simulink model "DconstI_snt"  (R2025b)
settings: Solver=ode45  StartTime=0.0  StopTime=10.0  RelTol=1e-3  EnableMultiTasking=on
undefined symbols (not defined in the file or in its folder): DiscIntNeverNeededParam, Ts
libraries: fl_lib x12, nesl_utility x12, mcbeeMathTransformLib x12, eeTransforms x12
settings Model: Creator=gdudgeon  LastModifiedBy=gdudgeon
settings SolverCC: AlgebraicLoopSolver=TrustRegion
settings DataIOCC: LimitDataPoints=on  SaveFormat=Array  ReturnWorkspaceOutputs=off
settings OptimizationCC: ExpressionDepthLimit=2147483647.0  LifeSpan=inf
settings DebuggingCC: UnderspecifiedInitializationDetection=Classic  MergeDetectMultiDrivingBlocksExec=none  SolverPrmCheckMsg=warning  UnconnectedInputMsg=warning  UnconnectedOutputMsg=warning  UnconnectedLineMsg=warning  StateNameClashWarn=warning  SFUnexpectedBacktrackingDiag=warning  SFNoUnconditionalDefaultTransitionDiag=warning  SFExecutionAtInitializationDiag=none  ArithmeticOperatorsInVariantConditions=warning
settings HardwareCC: ProdBitPerPointer=32.0  ProdBitPerSizeT=32.0  ProdBitPerPtrDiffT=32.0  ProdLargestAtomicFloat=None  ProdIntDivRoundTo=Undefined  ProdEndianess=Unspecified  ProdWordSize=32.0  ProdHWDeviceType=32-bit Generic
settings ModelReferenceCC: EnableRefExpFcnMdlSchedulingChecks=on  PropagateSignalLabelsOutOfModel=off
settings SFSimCC: SimUseLocalCustomCode=off  CustomCodeUndefinedFunction=UseInterfaceOnly
settings RTWCC: RTWUseLocalCustomCode=off  GPUComputeCapability=3.5
settings CodeAppCC: StateflowObjectComments=on
settings GRTTargetCC: TargetLangStandard=C89/C90 (ANSI)
settings ConfigComp: CovMetricSettings=dw  CovSaveCumulativeToWorkspaceVar=on  CovSaveSingleToWorkspaceVar=on  CovExternalEMLEnable=off  CovSFcnEnable=off
settings SimscapeCC: SimscapeNormalizeSystem=off

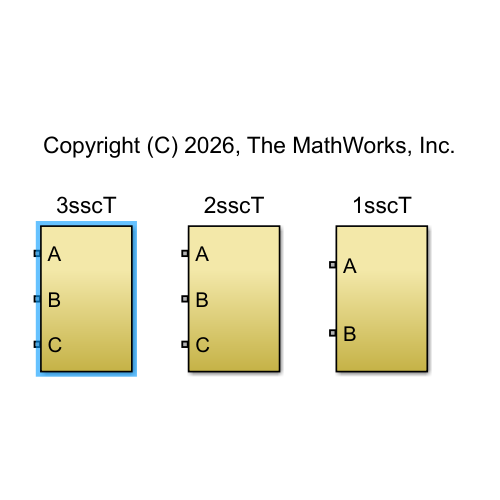
[thumbnail: Simulink's stored preview of the top-level diagram]
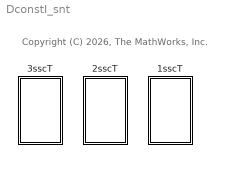
== system DconstI_snt ==
  note: Copyright (C) 2026, The MathWorks, Inc.
  1sscT : Subsystem
  2sscT : Subsystem
  3sscT : Subsystem

== system DconstI_snt/1sscT ==
  PQ1 : From
  constI1 : Subsystem  mask{V=4160*sqrt(2)}
      mask prompts: V "Vpk (V)"
  A : PMIOPort  Side=Left
  B : PMIOPort  Port=2  Side=Left
  wires:
  PQ1/1 -> constI1/1(PQ)
  connections:
  constI1/RConn1 -- A/RConn1
  constI1/LConn1 -- B/RConn1

== system DconstI_snt/2sscT ==
  PQ1 : From
  PQ2 : From
  constI1 : Subsystem  mask{V=4160*sqrt(2)}
      mask prompts: V "Vpk (V)"
  constI2 : Subsystem  mask{V=4160*sqrt(2)}
      mask prompts: V "Vpk (V)"
  A : PMIOPort  Side=Left
  B : PMIOPort  Port=2  Side=Left
  C : PMIOPort  Port=3  Side=Left
  wires:
  PQ2/1 -> constI2/1(PQ)
  PQ1/1 -> constI1/1(PQ)
  connections:
  constI2/LConn1 -- C/RConn1
  B/RConn1 -- constI2/RConn1 -- constI1/LConn1
  constI1/RConn1 -- A/RConn1

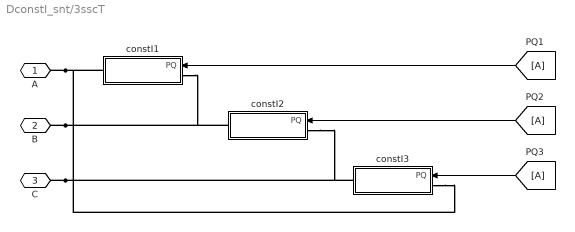
== system DconstI_snt/3sscT ==
  PQ1 : From
  PQ2 : From
  PQ3 : From
  constI1 : Subsystem  mask{V=4160*sqrt(2)}
      mask prompts: V "Vpk (V)"
  constI2 : Subsystem  mask{V=4160*sqrt(2)}
      mask prompts: V "Vpk (V)"
  constI3 : Subsystem  mask{V=4160*sqrt(2)}
      mask prompts: V "Vpk (V)"
  A : PMIOPort  Side=Left
  B : PMIOPort  Port=2  Side=Left
  C : PMIOPort  Port=3  Side=Left
  wires:
  PQ3/1 -> constI3/1(PQ)
  PQ1/1 -> constI1/1(PQ)
  PQ2/1 -> constI2/1(PQ)
  connections:
  A/RConn1 -- constI3/LConn1 -- constI1/RConn1
  B/RConn1 -- constI2/RConn1 -- constI1/LConn1
  C/RConn1 -- constI3/RConn1 -- constI2/LConn1

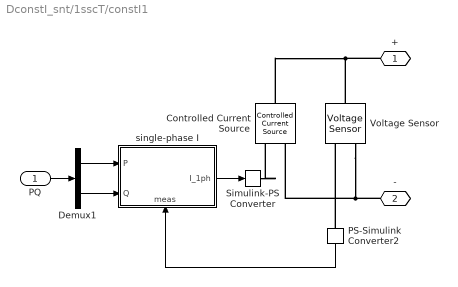
== system DconstI_snt/1sscT/constI1 ==
  PQ : Inport
  Controlled Current Source : fl_lib/Electrical/Electrical Sources/Controlled Current Source
  Demux1 : Demux  Outputs=2
  PS-Simulink Converter2 : nesl_utility/PS-Simulink Converter  PhysicalDomain=network_engine_domain  SubClassName=ps_output  LeftPortType=input  RightPortType=output  PseudoPeriodic=off  Frequencies=[]  VectorFormat=inherit  Unit=inherit  AffineConversion=off
  Simulink-PS Converter : nesl_utility/Simulink-PS Converter  PhysicalDomain=network_engine_domain  SubClassName=ps_input  LeftPortType=input  RightPortType=output  PseudoPeriodic=off  Frequencies=[]  NoiseDistribution=none  NoiseParameters=[]  Unit=1  AffineConversion=off  FilteringAndDerivatives=zero  SimscapeFilterOrder=1  InputFilterTimeConstant=0.001  UdotUserProvided=0
  Voltage Sensor : fl_lib/Electrical/Electrical Sensors/Voltage Sensor
  single-phase I : Subsystem
      settings: PortSchema="{\"entries\":[{\"content\":{\"sides\":[{\"content\":{\"connectorIds\":[\"In1\",\"In2\"]},\"type\":\"ConnectorPlacement.EquallySpacedRectSide\",\"uuid\":\"dcb77ad6-d65a-4afe-9b75-44cea2e03bc8\"},{\"content\":{\"connectorIds\":[\"Out1\"],\"side\":\"RIGHT\"},\"type\":\"ConnectorPlacement.EquallySpacedRectSide\",\"uuid\":\"20550ec8-912f-4e6b-8efc-55d7f6680ac4\"},{\"content\":{\"side\":\"TOP\"},\"type\":\"ConnectorPlacement.EquallySpacedRectSide\",\"uuid\":\"6ad8cbf4-1495-4620-97d9-4b8af34d00d1\"},{\"content\":{\"connectorIds\":[\"In3\"],\"side\":\"BOTTOM\"},\"type\":\"ConnectorPlacement.EquallySpacedRectSide\",\"uuid\":\"0b9a8788-8400-4a69-9d07-dd0028530e33\"}]},\"type\":\"ConnectorPlacement.EquallySpacedConnector\",\"uuid\":\"b57ec49b-aa32-43b3-a026-14ed90072d63\"}],\"packageUris\":[\"http://schema.mathworks.com/mf0/Connector/R2020b\"],\"version\":\"1.0\"}"
  + : PMIOPort  Side=Right
  - : PMIOPort  Port=2  Side=Left
  wires:
  single-phase I/1(I_1ph) -> Simulink-PS Converter/1
  Demux1/1 -> single-phase I/1(P)
  PQ/1 -> Demux1/1
  PS-Simulink Converter2/1 -> single-phase I/3(meas)
  Demux1/2 -> single-phase I/2(Q)
  connections:
  PS-Simulink Converter2/LConn1 -- Voltage Sensor/RConn1
  Simulink-PS Converter/RConn1 -- Controlled Current Source/RConn1
  -/RConn1 -- Controlled Current Source/RConn2 -- Voltage Sensor/RConn2
  +/RConn1 -- Controlled Current Source/LConn1 -- Voltage Sensor/LConn1

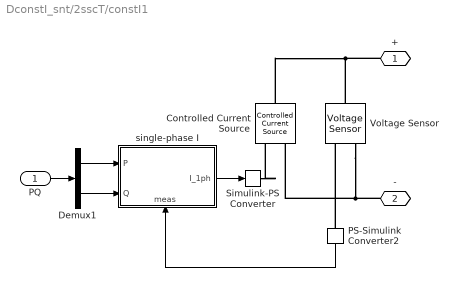
== system DconstI_snt/2sscT/constI1 ==
  PQ : Inport
  Controlled Current Source : fl_lib/Electrical/Electrical Sources/Controlled Current Source
  Demux1 : Demux  Outputs=2
  PS-Simulink Converter2 : nesl_utility/PS-Simulink Converter  PhysicalDomain=network_engine_domain  SubClassName=ps_output  LeftPortType=input  RightPortType=output  PseudoPeriodic=off  Frequencies=[]  VectorFormat=inherit  Unit=inherit  AffineConversion=off
  Simulink-PS Converter : nesl_utility/Simulink-PS Converter  PhysicalDomain=network_engine_domain  SubClassName=ps_input  LeftPortType=input  RightPortType=output  PseudoPeriodic=off  Frequencies=[]  NoiseDistribution=none  NoiseParameters=[]  Unit=1  AffineConversion=off  FilteringAndDerivatives=zero  SimscapeFilterOrder=1  InputFilterTimeConstant=0.001  UdotUserProvided=0
  Voltage Sensor : fl_lib/Electrical/Electrical Sensors/Voltage Sensor
  single-phase I : Subsystem
      settings: PortSchema="{\"entries\":[{\"content\":{\"sides\":[{\"content\":{\"connectorIds\":[\"In1\",\"In2\"]},\"type\":\"ConnectorPlacement.EquallySpacedRectSide\",\"uuid\":\"dcb77ad6-d65a-4afe-9b75-44cea2e03bc8\"},{\"content\":{\"connectorIds\":[\"Out1\"],\"side\":\"RIGHT\"},\"type\":\"ConnectorPlacement.EquallySpacedRectSide\",\"uuid\":\"20550ec8-912f-4e6b-8efc-55d7f6680ac4\"},{\"content\":{\"side\":\"TOP\"},\"type\":\"ConnectorPlacement.EquallySpacedRectSide\",\"uuid\":\"6ad8cbf4-1495-4620-97d9-4b8af34d00d1\"},{\"content\":{\"connectorIds\":[\"In3\"],\"side\":\"BOTTOM\"},\"type\":\"ConnectorPlacement.EquallySpacedRectSide\",\"uuid\":\"0b9a8788-8400-4a69-9d07-dd0028530e33\"}]},\"type\":\"ConnectorPlacement.EquallySpacedConnector\",\"uuid\":\"b57ec49b-aa32-43b3-a026-14ed90072d63\"}],\"packageUris\":[\"http://schema.mathworks.com/mf0/Connector/R2020b\"],\"version\":\"1.0\"}"
  + : PMIOPort  Side=Right
  - : PMIOPort  Port=2  Side=Left
  wires:
  single-phase I/1(I_1ph) -> Simulink-PS Converter/1
  Demux1/1 -> single-phase I/1(P)
  PQ/1 -> Demux1/1
  PS-Simulink Converter2/1 -> single-phase I/3(meas)
  Demux1/2 -> single-phase I/2(Q)
  connections:
  PS-Simulink Converter2/LConn1 -- Voltage Sensor/RConn1
  Simulink-PS Converter/RConn1 -- Controlled Current Source/RConn1
  -/RConn1 -- Controlled Current Source/RConn2 -- Voltage Sensor/RConn2
  +/RConn1 -- Controlled Current Source/LConn1 -- Voltage Sensor/LConn1

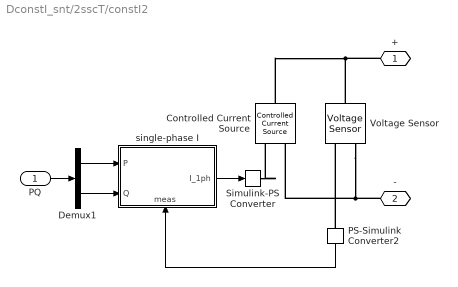
== system DconstI_snt/2sscT/constI2 ==
  PQ : Inport
  Controlled Current Source : fl_lib/Electrical/Electrical Sources/Controlled Current Source
  Demux1 : Demux  Outputs=2
  PS-Simulink Converter2 : nesl_utility/PS-Simulink Converter  PhysicalDomain=network_engine_domain  SubClassName=ps_output  LeftPortType=input  RightPortType=output  PseudoPeriodic=off  Frequencies=[]  VectorFormat=inherit  Unit=inherit  AffineConversion=off
  Simulink-PS Converter : nesl_utility/Simulink-PS Converter  PhysicalDomain=network_engine_domain  SubClassName=ps_input  LeftPortType=input  RightPortType=output  PseudoPeriodic=off  Frequencies=[]  NoiseDistribution=none  NoiseParameters=[]  Unit=1  AffineConversion=off  FilteringAndDerivatives=zero  SimscapeFilterOrder=1  InputFilterTimeConstant=0.001  UdotUserProvided=0
  Voltage Sensor : fl_lib/Electrical/Electrical Sensors/Voltage Sensor
  single-phase I : Subsystem
      settings: PortSchema="{\"entries\":[{\"content\":{\"sides\":[{\"content\":{\"connectorIds\":[\"In1\",\"In2\"]},\"type\":\"ConnectorPlacement.EquallySpacedRectSide\",\"uuid\":\"dcb77ad6-d65a-4afe-9b75-44cea2e03bc8\"},{\"content\":{\"connectorIds\":[\"Out1\"],\"side\":\"RIGHT\"},\"type\":\"ConnectorPlacement.EquallySpacedRectSide\",\"uuid\":\"20550ec8-912f-4e6b-8efc-55d7f6680ac4\"},{\"content\":{\"side\":\"TOP\"},\"type\":\"ConnectorPlacement.EquallySpacedRectSide\",\"uuid\":\"6ad8cbf4-1495-4620-97d9-4b8af34d00d1\"},{\"content\":{\"connectorIds\":[\"In3\"],\"side\":\"BOTTOM\"},\"type\":\"ConnectorPlacement.EquallySpacedRectSide\",\"uuid\":\"0b9a8788-8400-4a69-9d07-dd0028530e33\"}]},\"type\":\"ConnectorPlacement.EquallySpacedConnector\",\"uuid\":\"b57ec49b-aa32-43b3-a026-14ed90072d63\"}],\"packageUris\":[\"http://schema.mathworks.com/mf0/Connector/R2020b\"],\"version\":\"1.0\"}"
  + : PMIOPort  Side=Right
  - : PMIOPort  Port=2  Side=Left
  wires:
  Demux1/2 -> single-phase I/2(Q)
  PS-Simulink Converter2/1 -> single-phase I/3(meas)
  PQ/1 -> Demux1/1
  Demux1/1 -> single-phase I/1(P)
  single-phase I/1(I_1ph) -> Simulink-PS Converter/1
  connections:
  Voltage Sensor/LConn1 -- Controlled Current Source/LConn1 -- +/RConn1
  Voltage Sensor/RConn2 -- Controlled Current Source/RConn2 -- -/RConn1
  Simulink-PS Converter/RConn1 -- Controlled Current Source/RConn1
  PS-Simulink Converter2/LConn1 -- Voltage Sensor/RConn1

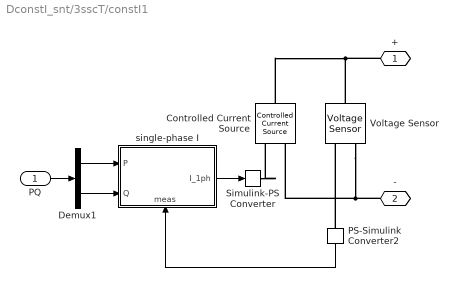
== system DconstI_snt/3sscT/constI1 ==
  PQ : Inport
  Controlled Current Source : fl_lib/Electrical/Electrical Sources/Controlled Current Source
  Demux1 : Demux  Outputs=2
  PS-Simulink Converter2 : nesl_utility/PS-Simulink Converter  PhysicalDomain=network_engine_domain  SubClassName=ps_output  LeftPortType=input  RightPortType=output  PseudoPeriodic=off  Frequencies=[]  VectorFormat=inherit  Unit=inherit  AffineConversion=off
  Simulink-PS Converter : nesl_utility/Simulink-PS Converter  PhysicalDomain=network_engine_domain  SubClassName=ps_input  LeftPortType=input  RightPortType=output  PseudoPeriodic=off  Frequencies=[]  NoiseDistribution=none  NoiseParameters=[]  Unit=1  AffineConversion=off  FilteringAndDerivatives=zero  SimscapeFilterOrder=1  InputFilterTimeConstant=0.001  UdotUserProvided=0
  Voltage Sensor : fl_lib/Electrical/Electrical Sensors/Voltage Sensor
  single-phase I : Subsystem
      settings: PortSchema="{\"entries\":[{\"content\":{\"sides\":[{\"content\":{\"connectorIds\":[\"In1\",\"In2\"]},\"type\":\"ConnectorPlacement.EquallySpacedRectSide\",\"uuid\":\"dcb77ad6-d65a-4afe-9b75-44cea2e03bc8\"},{\"content\":{\"connectorIds\":[\"Out1\"],\"side\":\"RIGHT\"},\"type\":\"ConnectorPlacement.EquallySpacedRectSide\",\"uuid\":\"20550ec8-912f-4e6b-8efc-55d7f6680ac4\"},{\"content\":{\"side\":\"TOP\"},\"type\":\"ConnectorPlacement.EquallySpacedRectSide\",\"uuid\":\"6ad8cbf4-1495-4620-97d9-4b8af34d00d1\"},{\"content\":{\"connectorIds\":[\"In3\"],\"side\":\"BOTTOM\"},\"type\":\"ConnectorPlacement.EquallySpacedRectSide\",\"uuid\":\"0b9a8788-8400-4a69-9d07-dd0028530e33\"}]},\"type\":\"ConnectorPlacement.EquallySpacedConnector\",\"uuid\":\"b57ec49b-aa32-43b3-a026-14ed90072d63\"}],\"packageUris\":[\"http://schema.mathworks.com/mf0/Connector/R2020b\"],\"version\":\"1.0\"}"
  + : PMIOPort  Side=Right
  - : PMIOPort  Port=2  Side=Left
  wires:
  single-phase I/1(I_1ph) -> Simulink-PS Converter/1
  Demux1/1 -> single-phase I/1(P)
  PQ/1 -> Demux1/1
  PS-Simulink Converter2/1 -> single-phase I/3(meas)
  Demux1/2 -> single-phase I/2(Q)
  connections:
  PS-Simulink Converter2/LConn1 -- Voltage Sensor/RConn1
  Simulink-PS Converter/RConn1 -- Controlled Current Source/RConn1
  -/RConn1 -- Controlled Current Source/RConn2 -- Voltage Sensor/RConn2
  +/RConn1 -- Controlled Current Source/LConn1 -- Voltage Sensor/LConn1

== system DconstI_snt/3sscT/constI2 ==
  PQ : Inport
  Controlled Current Source : fl_lib/Electrical/Electrical Sources/Controlled Current Source
  Demux1 : Demux  Outputs=2
  PS-Simulink Converter2 : nesl_utility/PS-Simulink Converter  PhysicalDomain=network_engine_domain  SubClassName=ps_output  LeftPortType=input  RightPortType=output  PseudoPeriodic=off  Frequencies=[]  VectorFormat=inherit  Unit=inherit  AffineConversion=off
  Simulink-PS Converter : nesl_utility/Simulink-PS Converter  PhysicalDomain=network_engine_domain  SubClassName=ps_input  LeftPortType=input  RightPortType=output  PseudoPeriodic=off  Frequencies=[]  NoiseDistribution=none  NoiseParameters=[]  Unit=1  AffineConversion=off  FilteringAndDerivatives=zero  SimscapeFilterOrder=1  InputFilterTimeConstant=0.001  UdotUserProvided=0
  Voltage Sensor : fl_lib/Electrical/Electrical Sensors/Voltage Sensor
  single-phase I : Subsystem
      settings: PortSchema="{\"entries\":[{\"content\":{\"sides\":[{\"content\":{\"connectorIds\":[\"In1\",\"In2\"]},\"type\":\"ConnectorPlacement.EquallySpacedRectSide\",\"uuid\":\"dcb77ad6-d65a-4afe-9b75-44cea2e03bc8\"},{\"content\":{\"connectorIds\":[\"Out1\"],\"side\":\"RIGHT\"},\"type\":\"ConnectorPlacement.EquallySpacedRectSide\",\"uuid\":\"20550ec8-912f-4e6b-8efc-55d7f6680ac4\"},{\"content\":{\"side\":\"TOP\"},\"type\":\"ConnectorPlacement.EquallySpacedRectSide\",\"uuid\":\"6ad8cbf4-1495-4620-97d9-4b8af34d00d1\"},{\"content\":{\"connectorIds\":[\"In3\"],\"side\":\"BOTTOM\"},\"type\":\"ConnectorPlacement.EquallySpacedRectSide\",\"uuid\":\"0b9a8788-8400-4a69-9d07-dd0028530e33\"}]},\"type\":\"ConnectorPlacement.EquallySpacedConnector\",\"uuid\":\"b57ec49b-aa32-43b3-a026-14ed90072d63\"}],\"packageUris\":[\"http://schema.mathworks.com/mf0/Connector/R2020b\"],\"version\":\"1.0\"}"
  + : PMIOPort  Side=Right
  - : PMIOPort  Port=2  Side=Left
  wires:
  Demux1/2 -> single-phase I/2(Q)
  PS-Simulink Converter2/1 -> single-phase I/3(meas)
  PQ/1 -> Demux1/1
  Demux1/1 -> single-phase I/1(P)
  single-phase I/1(I_1ph) -> Simulink-PS Converter/1
  connections:
  Voltage Sensor/LConn1 -- Controlled Current Source/LConn1 -- +/RConn1
  Voltage Sensor/RConn2 -- Controlled Current Source/RConn2 -- -/RConn1
  Simulink-PS Converter/RConn1 -- Controlled Current Source/RConn1
  PS-Simulink Converter2/LConn1 -- Voltage Sensor/RConn1

== system DconstI_snt/3sscT/constI3 ==
  PQ : Inport
  Controlled Current Source : fl_lib/Electrical/Electrical Sources/Controlled Current Source
  Demux1 : Demux  Outputs=2
  PS-Simulink Converter2 : nesl_utility/PS-Simulink Converter  PhysicalDomain=network_engine_domain  SubClassName=ps_output  LeftPortType=input  RightPortType=output  PseudoPeriodic=off  Frequencies=[]  VectorFormat=inherit  Unit=inherit  AffineConversion=off
  Simulink-PS Converter : nesl_utility/Simulink-PS Converter  PhysicalDomain=network_engine_domain  SubClassName=ps_input  LeftPortType=input  RightPortType=output  PseudoPeriodic=off  Frequencies=[]  NoiseDistribution=none  NoiseParameters=[]  Unit=1  AffineConversion=off  FilteringAndDerivatives=zero  SimscapeFilterOrder=1  InputFilterTimeConstant=0.001  UdotUserProvided=0
  Voltage Sensor : fl_lib/Electrical/Electrical Sensors/Voltage Sensor
  single-phase I : Subsystem
      settings: PortSchema="{\"entries\":[{\"content\":{\"sides\":[{\"content\":{\"connectorIds\":[\"In1\",\"In2\"]},\"type\":\"ConnectorPlacement.EquallySpacedRectSide\",\"uuid\":\"dcb77ad6-d65a-4afe-9b75-44cea2e03bc8\"},{\"content\":{\"connectorIds\":[\"Out1\"],\"side\":\"RIGHT\"},\"type\":\"ConnectorPlacement.EquallySpacedRectSide\",\"uuid\":\"20550ec8-912f-4e6b-8efc-55d7f6680ac4\"},{\"content\":{\"side\":\"TOP\"},\"type\":\"ConnectorPlacement.EquallySpacedRectSide\",\"uuid\":\"6ad8cbf4-1495-4620-97d9-4b8af34d00d1\"},{\"content\":{\"connectorIds\":[\"In3\"],\"side\":\"BOTTOM\"},\"type\":\"ConnectorPlacement.EquallySpacedRectSide\",\"uuid\":\"0b9a8788-8400-4a69-9d07-dd0028530e33\"}]},\"type\":\"ConnectorPlacement.EquallySpacedConnector\",\"uuid\":\"b57ec49b-aa32-43b3-a026-14ed90072d63\"}],\"packageUris\":[\"http://schema.mathworks.com/mf0/Connector/R2020b\"],\"version\":\"1.0\"}"
  + : PMIOPort  Side=Right
  - : PMIOPort  Port=2  Side=Left
  wires:
  single-phase I/1(I_1ph) -> Simulink-PS Converter/1
  Demux1/1 -> single-phase I/1(P)
  PQ/1 -> Demux1/1
  PS-Simulink Converter2/1 -> single-phase I/3(meas)
  Demux1/2 -> single-phase I/2(Q)
  connections:
  PS-Simulink Converter2/LConn1 -- Voltage Sensor/RConn1
  Simulink-PS Converter/RConn1 -- Controlled Current Source/RConn1
  -/RConn1 -- Controlled Current Source/RConn2 -- Voltage Sensor/RConn2
  +/RConn1 -- Controlled Current Source/LConn1 -- Voltage Sensor/LConn1

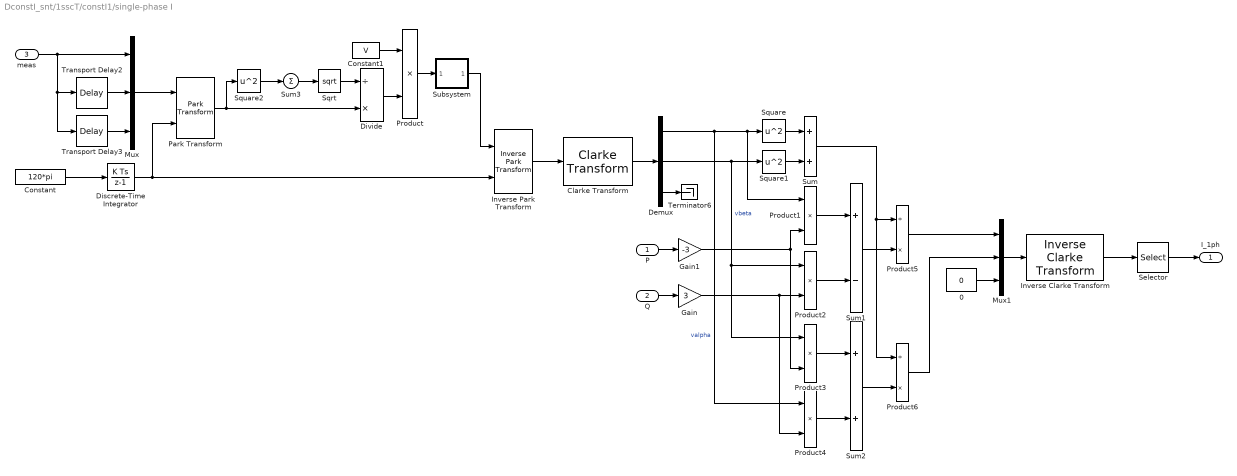
== system DconstI_snt/1sscT/constI1/single-phase I ==
  P : Inport
  Q : Inport  Port=2
  meas : Inport  Port=3
  "0 " : Constant  Value=0  VectorParams1D=off  SampleTime=Ts
  Clarke Transform : mcbeeMathTransformLib/Clarke Transform  PowerInvariant=on  UseWithEmbedded=off  PhaseInput=Two inputs
      settings: LibrarySourceBlock=|
      | ee_sl_lib/Mathematical
      | Transforms/Clarke Transform
  Constant : Constant  Value=120*pi  VectorParams1D=off  SampleTime=Ts
  Constant1 : Constant  Value=V  VectorParams1D=off  SampleTime=Ts
  Demux : Demux  Outputs=3
  Discrete-Time Integrator : DiscreteIntegrator  SampleTime=Ts  ICPrevOutput=DiscIntNeverNeededParam  ICPrevScaledInput=DiscIntNeverNeededParam
  Divide : Product  Inputs=/*
  Gain : Gain  Gain=3
  Gain1 : Gain  Gain=-3
  Inverse Clarke Transform : mcbeeMathTransformLib/Inverse Clarke Transform  PowerInvariant=on  UseWithEmbedded=off  PhaseInput=Two inputs
      settings: LibrarySourceBlock=|
      | ee_sl_lib/Mathematical
      | Transforms/Inverse
      | Clarke Transform
  Inverse Park Transform : eeTransforms/Inverse Park Transform  AxisAlignment=Q-axis  PowerInvariant=off
      settings: LibrarySourceBlock=|
      | ee_sl_lib/Mathematical
      | Transforms/Inverse
      | Park Transform
  Mux : Mux  Inputs=3
  Mux1 : Mux  Inputs=3
  Park Transform : eeTransforms/Park Transform  AxisAlignment=Q-axis  PowerInvariant=off
      settings: LibrarySourceBlock=|
      | ee_sl_lib/Mathematical
      | Transforms/Park Transform
  Product{,1..4} (5 alike) : Product
  Product5 : Product  Inputs=/*
  Product6 : Product  Inputs=/*
  Selector : Selector  InputPortWidth=3  IndexOptions=Index vector (dialog)  Indices=1  OutputSizes=1
  Sqrt : Sqrt
  Square : Math  Operator=square
  Square1 : Math  Operator=square
  Square2 : Math  Operator=square
  Subsystem : Subsystem
  Sum : Sum
  Sum1 : Sum  Inputs=+-
  Sum2 : Sum
  Sum3 : Sum  Inputs=+
  Terminator6 : Terminator
  Transport Delay2 : TransportDelay  DelayTime=1/180
  Transport Delay3 : TransportDelay  DelayTime=2/180
  I_1ph : Outport
  wires:
  Constant1/1 -> Product/1
  Sqrt/1 -> Divide/1
  Sum3/1 -> Sqrt/1
  Selector/1 -> I_1ph/1
  Mux/1 -> Park Transform/1
  Gain1/1 -> Product3/2, Product1/2
  Gain/1 -> Product2/2, Product4/2
  Transport Delay2/1 -> Mux/2
  meas/1 -> Mux/1, Transport Delay2/1, Transport Delay3/1
  Transport Delay3/1 -> Mux/3
  Discrete-Time Integrator/1 -> Park Transform/2, Inverse Park Transform/2
  Constant/1 -> Discrete-Time Integrator/1
  Product5/1 -> Mux1/1
  Square/1 -> Sum/1
  Product1/1 -> Sum1/1
  Product4/1 -> Sum2/2
  Product6/1 -> Mux1/2
  Demux/1 -> Square/1, Product1/1, Product4/1  "valpha"
  Product2/1 -> Sum1/2
  Sum1/1 -> Product5/2
  "0 "/1 -> Mux1/3
  Q/1 -> Gain/1
  Demux/2 -> Product2/1, Product3/1, Square1/1  "vbeta"
  Product3/1 -> Sum2/1
  Square1/1 -> Sum/2
  P/1 -> Gain1/1
  Sum/1 -> Product6/1, Product5/1
  Sum2/1 -> Product6/2
  Divide/1 -> Product/2
  Product/1 -> Subsystem/1(In1)
  Subsystem/1(Out1) -> Inverse Park Transform/1
  Park Transform/1 -> Square2/1, Divide/2
  Square2/1 -> Sum3/1
  Inverse Park Transform/1 -> Clarke Transform/1
  Clarke Transform/1 -> Demux/1
  Demux/3 -> Terminator6/1
  Mux1/1 -> Inverse Clarke Transform/1
  Inverse Clarke Transform/1 -> Selector/1

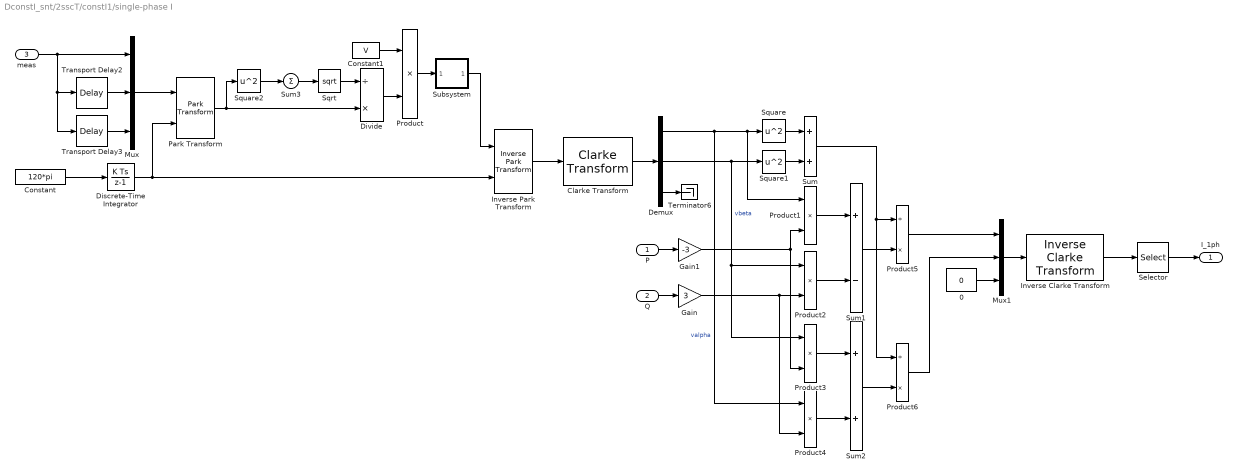
== system DconstI_snt/2sscT/constI1/single-phase I ==
  P : Inport
  Q : Inport  Port=2
  meas : Inport  Port=3
  "0 " : Constant  Value=0  VectorParams1D=off  SampleTime=Ts
  Clarke Transform : mcbeeMathTransformLib/Clarke Transform  PowerInvariant=on  UseWithEmbedded=off  PhaseInput=Two inputs
      settings: LibrarySourceBlock=|
      | ee_sl_lib/Mathematical
      | Transforms/Clarke Transform
  Constant : Constant  Value=120*pi  VectorParams1D=off  SampleTime=Ts
  Constant1 : Constant  Value=V  VectorParams1D=off  SampleTime=Ts
  Demux : Demux  Outputs=3
  Discrete-Time Integrator : DiscreteIntegrator  SampleTime=Ts  ICPrevOutput=DiscIntNeverNeededParam  ICPrevScaledInput=DiscIntNeverNeededParam
  Divide : Product  Inputs=/*
  Gain : Gain  Gain=3
  Gain1 : Gain  Gain=-3
  Inverse Clarke Transform : mcbeeMathTransformLib/Inverse Clarke Transform  PowerInvariant=on  UseWithEmbedded=off  PhaseInput=Two inputs
      settings: LibrarySourceBlock=|
      | ee_sl_lib/Mathematical
      | Transforms/Inverse
      | Clarke Transform
  Inverse Park Transform : eeTransforms/Inverse Park Transform  AxisAlignment=Q-axis  PowerInvariant=off
      settings: LibrarySourceBlock=|
      | ee_sl_lib/Mathematical
      | Transforms/Inverse
      | Park Transform
  Mux : Mux  Inputs=3
  Mux1 : Mux  Inputs=3
  Park Transform : eeTransforms/Park Transform  AxisAlignment=Q-axis  PowerInvariant=off
      settings: LibrarySourceBlock=|
      | ee_sl_lib/Mathematical
      | Transforms/Park Transform
  Product{,1..4} (5 alike) : Product
  Product5 : Product  Inputs=/*
  Product6 : Product  Inputs=/*
  Selector : Selector  InputPortWidth=3  IndexOptions=Index vector (dialog)  Indices=1  OutputSizes=1
  Sqrt : Sqrt
  Square : Math  Operator=square
  Square1 : Math  Operator=square
  Square2 : Math  Operator=square
  Subsystem : Subsystem
  Sum : Sum
  Sum1 : Sum  Inputs=+-
  Sum2 : Sum
  Sum3 : Sum  Inputs=+
  Terminator6 : Terminator
  Transport Delay2 : TransportDelay  DelayTime=1/180
  Transport Delay3 : TransportDelay  DelayTime=2/180
  I_1ph : Outport
  wires:
  Constant1/1 -> Product/1
  Sqrt/1 -> Divide/1
  Sum3/1 -> Sqrt/1
  Selector/1 -> I_1ph/1
  Mux/1 -> Park Transform/1
  Gain1/1 -> Product3/2, Product1/2
  Gain/1 -> Product2/2, Product4/2
  Transport Delay2/1 -> Mux/2
  meas/1 -> Mux/1, Transport Delay2/1, Transport Delay3/1
  Transport Delay3/1 -> Mux/3
  Discrete-Time Integrator/1 -> Park Transform/2, Inverse Park Transform/2
  Constant/1 -> Discrete-Time Integrator/1
  Product5/1 -> Mux1/1
  Square/1 -> Sum/1
  Product1/1 -> Sum1/1
  Product4/1 -> Sum2/2
  Product6/1 -> Mux1/2
  Demux/1 -> Square/1, Product1/1, Product4/1  "valpha"
  Product2/1 -> Sum1/2
  Sum1/1 -> Product5/2
  "0 "/1 -> Mux1/3
  Q/1 -> Gain/1
  Demux/2 -> Product2/1, Product3/1, Square1/1  "vbeta"
  Product3/1 -> Sum2/1
  Square1/1 -> Sum/2
  P/1 -> Gain1/1
  Sum/1 -> Product6/1, Product5/1
  Sum2/1 -> Product6/2
  Divide/1 -> Product/2
  Product/1 -> Subsystem/1(In1)
  Subsystem/1(Out1) -> Inverse Park Transform/1
  Park Transform/1 -> Square2/1, Divide/2
  Square2/1 -> Sum3/1
  Inverse Park Transform/1 -> Clarke Transform/1
  Clarke Transform/1 -> Demux/1
  Demux/3 -> Terminator6/1
  Mux1/1 -> Inverse Clarke Transform/1
  Inverse Clarke Transform/1 -> Selector/1

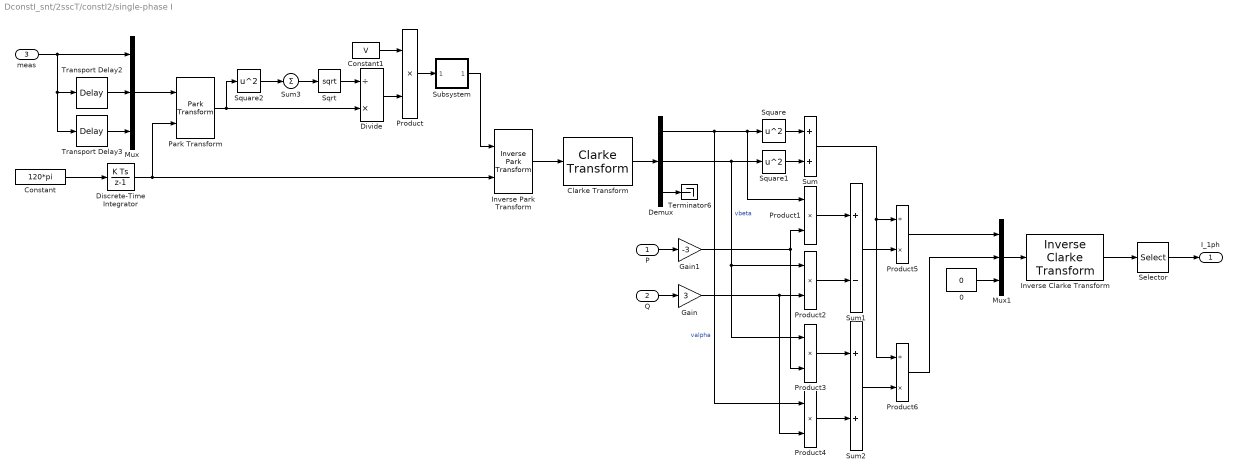
== system DconstI_snt/2sscT/constI2/single-phase I ==
  P : Inport
  Q : Inport  Port=2
  meas : Inport  Port=3
  "0 " : Constant  Value=0  VectorParams1D=off  SampleTime=Ts
  Clarke Transform : mcbeeMathTransformLib/Clarke Transform  PowerInvariant=on  UseWithEmbedded=off  PhaseInput=Two inputs
      settings: LibrarySourceBlock=|
      | ee_sl_lib/Mathematical
      | Transforms/Clarke Transform
  Constant : Constant  Value=120*pi  VectorParams1D=off  SampleTime=Ts
  Constant1 : Constant  Value=V  VectorParams1D=off  SampleTime=Ts
  Demux : Demux  Outputs=3
  Discrete-Time Integrator : DiscreteIntegrator  SampleTime=Ts  ICPrevOutput=DiscIntNeverNeededParam  ICPrevScaledInput=DiscIntNeverNeededParam
  Divide : Product  Inputs=/*
  Gain : Gain  Gain=3
  Gain1 : Gain  Gain=-3
  Inverse Clarke Transform : mcbeeMathTransformLib/Inverse Clarke Transform  PowerInvariant=on  UseWithEmbedded=off  PhaseInput=Two inputs
      settings: LibrarySourceBlock=|
      | ee_sl_lib/Mathematical
      | Transforms/Inverse
      | Clarke Transform
  Inverse Park Transform : eeTransforms/Inverse Park Transform  AxisAlignment=Q-axis  PowerInvariant=off
      settings: LibrarySourceBlock=|
      | ee_sl_lib/Mathematical
      | Transforms/Inverse
      | Park Transform
  Mux : Mux  Inputs=3
  Mux1 : Mux  Inputs=3
  Park Transform : eeTransforms/Park Transform  AxisAlignment=Q-axis  PowerInvariant=off
      settings: LibrarySourceBlock=|
      | ee_sl_lib/Mathematical
      | Transforms/Park Transform
  Product{,1..4} (5 alike) : Product
  Product5 : Product  Inputs=/*
  Product6 : Product  Inputs=/*
  Selector : Selector  InputPortWidth=3  IndexOptions=Index vector (dialog)  Indices=1  OutputSizes=1
  Sqrt : Sqrt
  Square : Math  Operator=square
  Square1 : Math  Operator=square
  Square2 : Math  Operator=square
  Subsystem : Subsystem
  Sum : Sum
  Sum1 : Sum  Inputs=+-
  Sum2 : Sum
  Sum3 : Sum  Inputs=+
  Terminator6 : Terminator
  Transport Delay2 : TransportDelay  DelayTime=1/180
  Transport Delay3 : TransportDelay  DelayTime=2/180
  I_1ph : Outport
  wires:
  Inverse Clarke Transform/1 -> Selector/1
  Mux1/1 -> Inverse Clarke Transform/1
  Demux/3 -> Terminator6/1
  Clarke Transform/1 -> Demux/1
  Inverse Park Transform/1 -> Clarke Transform/1
  Square2/1 -> Sum3/1
  Park Transform/1 -> Divide/2, Square2/1
  Subsystem/1(Out1) -> Inverse Park Transform/1
  Product/1 -> Subsystem/1(In1)
  Divide/1 -> Product/2
  Sum2/1 -> Product6/2
  Sum/1 -> Product5/1, Product6/1
  P/1 -> Gain1/1
  Square1/1 -> Sum/2
  Product3/1 -> Sum2/1
  Demux/2 -> Square1/1, Product3/1, Product2/1  "vbeta"
  Q/1 -> Gain/1
  "0 "/1 -> Mux1/3
  Sum1/1 -> Product5/2
  Product2/1 -> Sum1/2
  Demux/1 -> Product4/1, Product1/1, Square/1  "valpha"
  Product6/1 -> Mux1/2
  Product4/1 -> Sum2/2
  Product1/1 -> Sum1/1
  Square/1 -> Sum/1
  Product5/1 -> Mux1/1
  Constant/1 -> Discrete-Time Integrator/1
  Discrete-Time Integrator/1 -> Inverse Park Transform/2, Park Transform/2
  Transport Delay3/1 -> Mux/3
  meas/1 -> Transport Delay3/1, Transport Delay2/1, Mux/1
  Transport Delay2/1 -> Mux/2
  Gain/1 -> Product4/2, Product2/2
  Gain1/1 -> Product1/2, Product3/2
  Mux/1 -> Park Transform/1
  Selector/1 -> I_1ph/1
  Sum3/1 -> Sqrt/1
  Sqrt/1 -> Divide/1
  Constant1/1 -> Product/1

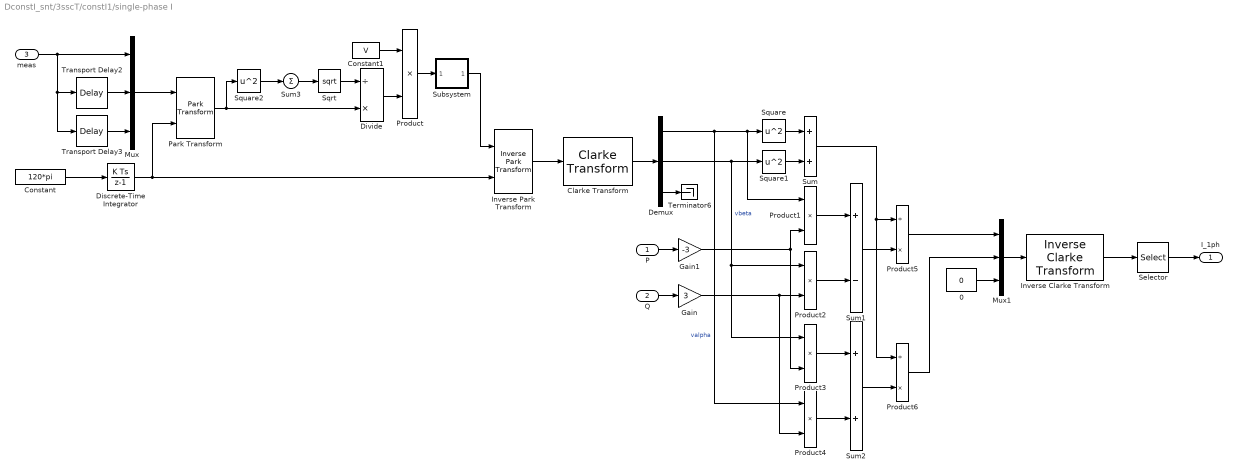
== system DconstI_snt/3sscT/constI1/single-phase I ==
  P : Inport
  Q : Inport  Port=2
  meas : Inport  Port=3
  "0 " : Constant  Value=0  VectorParams1D=off  SampleTime=Ts
  Clarke Transform : mcbeeMathTransformLib/Clarke Transform  PowerInvariant=on  UseWithEmbedded=off  PhaseInput=Two inputs
      settings: LibrarySourceBlock=|
      | ee_sl_lib/Mathematical
      | Transforms/Clarke Transform
  Constant : Constant  Value=120*pi  VectorParams1D=off  SampleTime=Ts
  Constant1 : Constant  Value=V  VectorParams1D=off  SampleTime=Ts
  Demux : Demux  Outputs=3
  Discrete-Time Integrator : DiscreteIntegrator  SampleTime=Ts  ICPrevOutput=DiscIntNeverNeededParam  ICPrevScaledInput=DiscIntNeverNeededParam
  Divide : Product  Inputs=/*
  Gain : Gain  Gain=3
  Gain1 : Gain  Gain=-3
  Inverse Clarke Transform : mcbeeMathTransformLib/Inverse Clarke Transform  PowerInvariant=on  UseWithEmbedded=off  PhaseInput=Two inputs
      settings: LibrarySourceBlock=|
      | ee_sl_lib/Mathematical
      | Transforms/Inverse
      | Clarke Transform
  Inverse Park Transform : eeTransforms/Inverse Park Transform  AxisAlignment=Q-axis  PowerInvariant=off
      settings: LibrarySourceBlock=|
      | ee_sl_lib/Mathematical
      | Transforms/Inverse
      | Park Transform
  Mux : Mux  Inputs=3
  Mux1 : Mux  Inputs=3
  Park Transform : eeTransforms/Park Transform  AxisAlignment=Q-axis  PowerInvariant=off
      settings: LibrarySourceBlock=|
      | ee_sl_lib/Mathematical
      | Transforms/Park Transform
  Product{,1..4} (5 alike) : Product
  Product5 : Product  Inputs=/*
  Product6 : Product  Inputs=/*
  Selector : Selector  InputPortWidth=3  IndexOptions=Index vector (dialog)  Indices=1  OutputSizes=1
  Sqrt : Sqrt
  Square : Math  Operator=square
  Square1 : Math  Operator=square
  Square2 : Math  Operator=square
  Subsystem : Subsystem
  Sum : Sum
  Sum1 : Sum  Inputs=+-
  Sum2 : Sum
  Sum3 : Sum  Inputs=+
  Terminator6 : Terminator
  Transport Delay2 : TransportDelay  DelayTime=1/180
  Transport Delay3 : TransportDelay  DelayTime=2/180
  I_1ph : Outport
  wires:
  Constant1/1 -> Product/1
  Sqrt/1 -> Divide/1
  Sum3/1 -> Sqrt/1
  Selector/1 -> I_1ph/1
  Mux/1 -> Park Transform/1
  Gain1/1 -> Product3/2, Product1/2
  Gain/1 -> Product2/2, Product4/2
  Transport Delay2/1 -> Mux/2
  meas/1 -> Mux/1, Transport Delay2/1, Transport Delay3/1
  Transport Delay3/1 -> Mux/3
  Discrete-Time Integrator/1 -> Park Transform/2, Inverse Park Transform/2
  Constant/1 -> Discrete-Time Integrator/1
  Product5/1 -> Mux1/1
  Square/1 -> Sum/1
  Product1/1 -> Sum1/1
  Product4/1 -> Sum2/2
  Product6/1 -> Mux1/2
  Demux/1 -> Square/1, Product1/1, Product4/1  "valpha"
  Product2/1 -> Sum1/2
  Sum1/1 -> Product5/2
  "0 "/1 -> Mux1/3
  Q/1 -> Gain/1
  Demux/2 -> Product2/1, Product3/1, Square1/1  "vbeta"
  Product3/1 -> Sum2/1
  Square1/1 -> Sum/2
  P/1 -> Gain1/1
  Sum/1 -> Product6/1, Product5/1
  Sum2/1 -> Product6/2
  Divide/1 -> Product/2
  Product/1 -> Subsystem/1(In1)
  Subsystem/1(Out1) -> Inverse Park Transform/1
  Park Transform/1 -> Square2/1, Divide/2
  Square2/1 -> Sum3/1
  Inverse Park Transform/1 -> Clarke Transform/1
  Clarke Transform/1 -> Demux/1
  Demux/3 -> Terminator6/1
  Mux1/1 -> Inverse Clarke Transform/1
  Inverse Clarke Transform/1 -> Selector/1

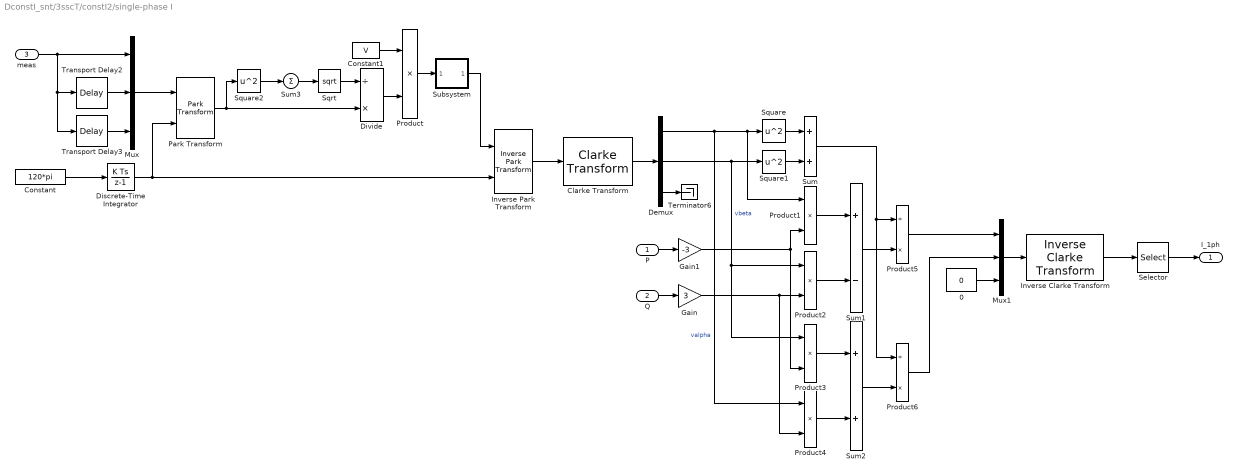
== system DconstI_snt/3sscT/constI2/single-phase I ==
  P : Inport
  Q : Inport  Port=2
  meas : Inport  Port=3
  "0 " : Constant  Value=0  VectorParams1D=off  SampleTime=Ts
  Clarke Transform : mcbeeMathTransformLib/Clarke Transform  PowerInvariant=on  UseWithEmbedded=off  PhaseInput=Two inputs
      settings: LibrarySourceBlock=|
      | ee_sl_lib/Mathematical
      | Transforms/Clarke Transform
  Constant : Constant  Value=120*pi  VectorParams1D=off  SampleTime=Ts
  Constant1 : Constant  Value=V  VectorParams1D=off  SampleTime=Ts
  Demux : Demux  Outputs=3
  Discrete-Time Integrator : DiscreteIntegrator  SampleTime=Ts  ICPrevOutput=DiscIntNeverNeededParam  ICPrevScaledInput=DiscIntNeverNeededParam
  Divide : Product  Inputs=/*
  Gain : Gain  Gain=3
  Gain1 : Gain  Gain=-3
  Inverse Clarke Transform : mcbeeMathTransformLib/Inverse Clarke Transform  PowerInvariant=on  UseWithEmbedded=off  PhaseInput=Two inputs
      settings: LibrarySourceBlock=|
      | ee_sl_lib/Mathematical
      | Transforms/Inverse
      | Clarke Transform
  Inverse Park Transform : eeTransforms/Inverse Park Transform  AxisAlignment=Q-axis  PowerInvariant=off
      settings: LibrarySourceBlock=|
      | ee_sl_lib/Mathematical
      | Transforms/Inverse
      | Park Transform
  Mux : Mux  Inputs=3
  Mux1 : Mux  Inputs=3
  Park Transform : eeTransforms/Park Transform  AxisAlignment=Q-axis  PowerInvariant=off
      settings: LibrarySourceBlock=|
      | ee_sl_lib/Mathematical
      | Transforms/Park Transform
  Product{,1..4} (5 alike) : Product
  Product5 : Product  Inputs=/*
  Product6 : Product  Inputs=/*
  Selector : Selector  InputPortWidth=3  IndexOptions=Index vector (dialog)  Indices=1  OutputSizes=1
  Sqrt : Sqrt
  Square : Math  Operator=square
  Square1 : Math  Operator=square
  Square2 : Math  Operator=square
  Subsystem : Subsystem
  Sum : Sum
  Sum1 : Sum  Inputs=+-
  Sum2 : Sum
  Sum3 : Sum  Inputs=+
  Terminator6 : Terminator
  Transport Delay2 : TransportDelay  DelayTime=1/180
  Transport Delay3 : TransportDelay  DelayTime=2/180
  I_1ph : Outport
  wires:
  Inverse Clarke Transform/1 -> Selector/1
  Mux1/1 -> Inverse Clarke Transform/1
  Demux/3 -> Terminator6/1
  Clarke Transform/1 -> Demux/1
  Inverse Park Transform/1 -> Clarke Transform/1
  Square2/1 -> Sum3/1
  Park Transform/1 -> Divide/2, Square2/1
  Subsystem/1(Out1) -> Inverse Park Transform/1
  Product/1 -> Subsystem/1(In1)
  Divide/1 -> Product/2
  Sum2/1 -> Product6/2
  Sum/1 -> Product5/1, Product6/1
  P/1 -> Gain1/1
  Square1/1 -> Sum/2
  Product3/1 -> Sum2/1
  Demux/2 -> Square1/1, Product3/1, Product2/1  "vbeta"
  Q/1 -> Gain/1
  "0 "/1 -> Mux1/3
  Sum1/1 -> Product5/2
  Product2/1 -> Sum1/2
  Demux/1 -> Product4/1, Product1/1, Square/1  "valpha"
  Product6/1 -> Mux1/2
  Product4/1 -> Sum2/2
  Product1/1 -> Sum1/1
  Square/1 -> Sum/1
  Product5/1 -> Mux1/1
  Constant/1 -> Discrete-Time Integrator/1
  Discrete-Time Integrator/1 -> Inverse Park Transform/2, Park Transform/2
  Transport Delay3/1 -> Mux/3
  meas/1 -> Transport Delay3/1, Transport Delay2/1, Mux/1
  Transport Delay2/1 -> Mux/2
  Gain/1 -> Product4/2, Product2/2
  Gain1/1 -> Product1/2, Product3/2
  Mux/1 -> Park Transform/1
  Selector/1 -> I_1ph/1
  Sum3/1 -> Sqrt/1
  Sqrt/1 -> Divide/1
  Constant1/1 -> Product/1

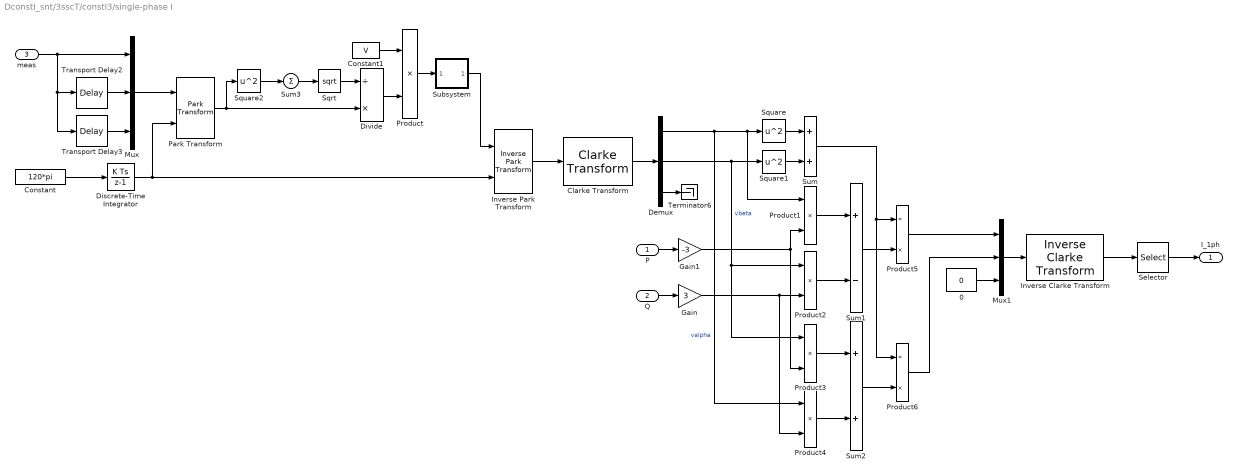
== system DconstI_snt/3sscT/constI3/single-phase I ==
  P : Inport
  Q : Inport  Port=2
  meas : Inport  Port=3
  "0 " : Constant  Value=0  VectorParams1D=off  SampleTime=Ts
  Clarke Transform : mcbeeMathTransformLib/Clarke Transform  PowerInvariant=on  UseWithEmbedded=off  PhaseInput=Two inputs
      settings: LibrarySourceBlock=|
      | ee_sl_lib/Mathematical
      | Transforms/Clarke Transform
  Constant : Constant  Value=120*pi  VectorParams1D=off  SampleTime=Ts
  Constant1 : Constant  Value=V  VectorParams1D=off  SampleTime=Ts
  Demux : Demux  Outputs=3
  Discrete-Time Integrator : DiscreteIntegrator  SampleTime=Ts  ICPrevOutput=DiscIntNeverNeededParam  ICPrevScaledInput=DiscIntNeverNeededParam
  Divide : Product  Inputs=/*
  Gain : Gain  Gain=3
  Gain1 : Gain  Gain=-3
  Inverse Clarke Transform : mcbeeMathTransformLib/Inverse Clarke Transform  PowerInvariant=on  UseWithEmbedded=off  PhaseInput=Two inputs
      settings: LibrarySourceBlock=|
      | ee_sl_lib/Mathematical
      | Transforms/Inverse
      | Clarke Transform
  Inverse Park Transform : eeTransforms/Inverse Park Transform  AxisAlignment=Q-axis  PowerInvariant=off
      settings: LibrarySourceBlock=|
      | ee_sl_lib/Mathematical
      | Transforms/Inverse
      | Park Transform
  Mux : Mux  Inputs=3
  Mux1 : Mux  Inputs=3
  Park Transform : eeTransforms/Park Transform  AxisAlignment=Q-axis  PowerInvariant=off
      settings: LibrarySourceBlock=|
      | ee_sl_lib/Mathematical
      | Transforms/Park Transform
  Product{,1..4} (5 alike) : Product
  Product5 : Product  Inputs=/*
  Product6 : Product  Inputs=/*
  Selector : Selector  InputPortWidth=3  IndexOptions=Index vector (dialog)  Indices=1  OutputSizes=1
  Sqrt : Sqrt
  Square : Math  Operator=square
  Square1 : Math  Operator=square
  Square2 : Math  Operator=square
  Subsystem : Subsystem
  Sum : Sum
  Sum1 : Sum  Inputs=+-
  Sum2 : Sum
  Sum3 : Sum  Inputs=+
  Terminator6 : Terminator
  Transport Delay2 : TransportDelay  DelayTime=1/180
  Transport Delay3 : TransportDelay  DelayTime=2/180
  I_1ph : Outport
  wires:
  Constant1/1 -> Product/1
  Sqrt/1 -> Divide/1
  Sum3/1 -> Sqrt/1
  Selector/1 -> I_1ph/1
  Mux/1 -> Park Transform/1
  Gain1/1 -> Product3/2, Product1/2
  Gain/1 -> Product2/2, Product4/2
  Transport Delay2/1 -> Mux/2
  meas/1 -> Mux/1, Transport Delay2/1, Transport Delay3/1
  Transport Delay3/1 -> Mux/3
  Discrete-Time Integrator/1 -> Park Transform/2, Inverse Park Transform/2
  Constant/1 -> Discrete-Time Integrator/1
  Product5/1 -> Mux1/1
  Square/1 -> Sum/1
  Product1/1 -> Sum1/1
  Product4/1 -> Sum2/2
  Product6/1 -> Mux1/2
  Demux/1 -> Square/1, Product1/1, Product4/1  "valpha"
  Product2/1 -> Sum1/2
  Sum1/1 -> Product5/2
  "0 "/1 -> Mux1/3
  Q/1 -> Gain/1
  Demux/2 -> Product2/1, Product3/1, Square1/1  "vbeta"
  Product3/1 -> Sum2/1
  Square1/1 -> Sum/2
  P/1 -> Gain1/1
  Sum/1 -> Product6/1, Product5/1
  Sum2/1 -> Product6/2
  Divide/1 -> Product/2
  Product/1 -> Subsystem/1(In1)
  Subsystem/1(Out1) -> Inverse Park Transform/1
  Park Transform/1 -> Square2/1, Divide/2
  Square2/1 -> Sum3/1
  Inverse Park Transform/1 -> Clarke Transform/1
  Clarke Transform/1 -> Demux/1
  Demux/3 -> Terminator6/1
  Mux1/1 -> Inverse Clarke Transform/1
  Inverse Clarke Transform/1 -> Selector/1

== system DconstI_snt/1sscT/constI1/single-phase I/Subsystem ==
  In1 : Inport
  Discrete-Time Integrator : DiscreteIntegrator  gainval=1/Ts/20  InitialCondition=2000  SampleTime=-1  ICPrevOutput=DiscIntNeverNeededParam  ICPrevScaledInput=DiscIntNeverNeededParam
  Sum : Sum  Inputs=|+-
  Out1 : Outport
  wires:
  Discrete-Time Integrator/1 -> Out1/1, Sum/2
  Sum/1 -> Discrete-Time Integrator/1
  In1/1 -> Sum/1

== system DconstI_snt/2sscT/constI1/single-phase I/Subsystem ==
  In1 : Inport
  Discrete-Time Integrator : DiscreteIntegrator  gainval=1/Ts/20  InitialCondition=2000  SampleTime=-1  ICPrevOutput=DiscIntNeverNeededParam  ICPrevScaledInput=DiscIntNeverNeededParam
  Sum : Sum  Inputs=|+-
  Out1 : Outport
  wires:
  Discrete-Time Integrator/1 -> Out1/1, Sum/2
  Sum/1 -> Discrete-Time Integrator/1
  In1/1 -> Sum/1

== system DconstI_snt/2sscT/constI2/single-phase I/Subsystem ==
  In1 : Inport
  Discrete-Time Integrator : DiscreteIntegrator  gainval=1/Ts/20  InitialCondition=2000  SampleTime=-1  ICPrevOutput=DiscIntNeverNeededParam  ICPrevScaledInput=DiscIntNeverNeededParam
  Sum : Sum  Inputs=|+-
  Out1 : Outport
  wires:
  In1/1 -> Sum/1
  Sum/1 -> Discrete-Time Integrator/1
  Discrete-Time Integrator/1 -> Sum/2, Out1/1

== system DconstI_snt/3sscT/constI1/single-phase I/Subsystem ==
  In1 : Inport
  Discrete-Time Integrator : DiscreteIntegrator  gainval=1/Ts/20  InitialCondition=2000  SampleTime=-1  ICPrevOutput=DiscIntNeverNeededParam  ICPrevScaledInput=DiscIntNeverNeededParam
  Sum : Sum  Inputs=|+-
  Out1 : Outport
  wires:
  Discrete-Time Integrator/1 -> Out1/1, Sum/2
  Sum/1 -> Discrete-Time Integrator/1
  In1/1 -> Sum/1

== system DconstI_snt/3sscT/constI2/single-phase I/Subsystem ==
  In1 : Inport
  Discrete-Time Integrator : DiscreteIntegrator  gainval=1/Ts/20  InitialCondition=2000  SampleTime=-1  ICPrevOutput=DiscIntNeverNeededParam  ICPrevScaledInput=DiscIntNeverNeededParam
  Sum : Sum  Inputs=|+-
  Out1 : Outport
  wires:
  In1/1 -> Sum/1
  Sum/1 -> Discrete-Time Integrator/1
  Discrete-Time Integrator/1 -> Sum/2, Out1/1

== system DconstI_snt/3sscT/constI3/single-phase I/Subsystem ==
  In1 : Inport
  Discrete-Time Integrator : DiscreteIntegrator  gainval=1/Ts/20  InitialCondition=2000  SampleTime=-1  ICPrevOutput=DiscIntNeverNeededParam  ICPrevScaledInput=DiscIntNeverNeededParam
  Sum : Sum  Inputs=|+-
  Out1 : Outport
  wires:
  Discrete-Time Integrator/1 -> Out1/1, Sum/2
  Sum/1 -> Discrete-Time Integrator/1
  In1/1 -> Sum/1
